simulink model "game"  (R2021a)
settings: Solver=VariableStepAuto  StartTime=0.0  StopTime=inf  RelTol=1e-3
libraries: vrlib x2
settings Model: Creator=kbhar  LastModifiedBy=kbhar

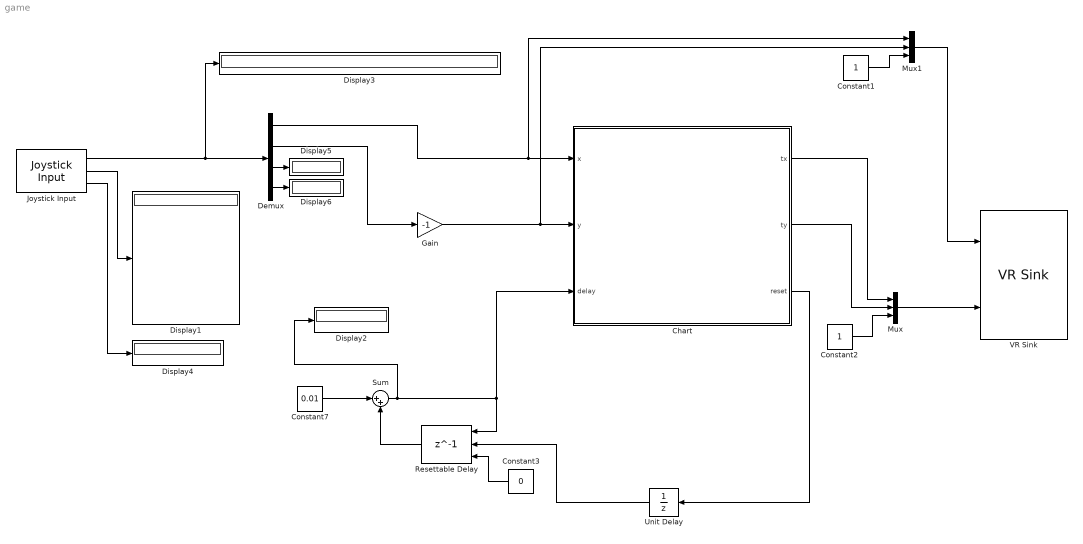
== system game ==
  Chart : Stateflow chart  TreatAsAtomicUnit=on
      settings: PortSchema="{\"entries\":[{\"content\":{\"sides\":[{\"content\":{\"connectorIds\":[\"In2\",\"In3\",\"In1\"]},\"type\":\"ConnectorPlacement.EquallySpacedRectSide\",\"uuid\":\"f1ac4276-d975-44f7-8e33-a85bf0c84183\"},{\"content\":{\"connectorIds\":[\"Out1\",\"Out2\",\"Out3\"],\"side\":\"RIGHT\"},\"type\":\"ConnectorPlacement.EquallySpacedRectSide\",\"uuid\":\"fad27161-645b-4edf-96e2-08eec94c36d6\"},{\"content\":{\"connectorIds\":[],\"side\":\"TOP\"},\"type\":\"ConnectorPlacement.EquallySpacedRectSide\",\"uuid\":\"b77dfb51-8030-4063-824e-9da8b3bcfc4a\"}]},\"type\":\"ConnectorPlacement.EquallySpacedConnector\",\"uuid\":\"85b5c07b-9026-46b4-be3f-3c9b0e47e395\"}],\"packageUris\":[\"http://schema.mathworks.com/mf0/Connector/R2020b\"],\"version\":\"1.0\"}"
  Constant1 : Constant
  Constant2 : Constant
  Constant3 : Constant  Value=0
  Constant7 : Constant  Value=0.01
  Demux : Demux
  Display{1..6} (6 alike) : Display
  Gain : Gain  Gain=-1
  Joystick Input : vrlib/Joystick Input  joyid=1  adjustports=on  forcefeed=off
  Mux : Mux  Inputs=3
  Mux1 : Mux  Inputs=3
  Resettable Delay : Delay  DelayLength=1  InitialConditionSource=Input port  ExternalReset=Rising
      settings: InputPortMap=u0,r5,p4
  Sum : Sum  Inputs=|++
  Unit Delay : UnitDelay  SampleTime=-1  HasFrameUpgradeWarning=on
  VR Sink : vrlib/VR Sink  InstantiateOnLoad=on  SampleTime=0.1  ViewEnable=on  RemoteChange=off  RemoteView=off  FieldsWritten=cursor.translation.3.1.1.double#target.translation.3.1.1.double  WorldFileName=game.wrl  AutoView=off  VideoDimensions=[]  AllowVariableSize=off  FigureProperties="{'Position', 'Name', 'Viewpoint', 'CameraBound', 'CameraDirection', 'CameraPosition', 'CameraUpVector', 'ZoomFactor', 'Antialiasing', 'Headlight', 'Lighting', 'NavPanel', 'Sound', 'StatusBar', 'Stereo3D', 'Stereo3DCameraOffset', 'Stereo3DHIT', 'ToolBar', 'Textures', 'Transparency', 'Triad', 'Wireframe', 'NavZones', 'NavMode', 'NavSpeed', 'CaptureFileFormat', 'CaptureFileName', 'Record2DCompressMethod', 'Record2DCompressQuality', 'Record2D', 'Record2DFileName', 'Record2DFPS'; [7.8340000000000009e+02   2.7179999999999995e+02   5.7600000000000000e+02   3.5000000000000000e+02], '', '', 'on', [-1.1111111570273457e-04   0.0000000000000000e+00  -9.9999999382716009e-01], [-2.1809524624175411e-04   5.2244997024536133e-01   8.0371428770549223e+00], [0.0000000000000000e+00   1.0000000000000000e+00   0.0000000000000000e+00], [1.0000000000000000e+00], 'on', 'on', 'on', 'halfbar', 'on', 'on', 'off', [1.0000000149011612e-01], [0.0000000000000000e+00], 'on', 'on', 'on', 'none', 'off', 'off', 'fly', 'normal', 'tif', '%f_anim_%n.tif', 'auto', [7.5000000000000000e+01], 'off', '%f_anim_%n.avi', 'auto'}"
  wires:
  Resettable Delay/1 -> Sum/2
  Constant7/1 -> Sum/1
  Sum/1 -> Display2/1, Resettable Delay/1, Chart/1(delay)
  Chart/3(reset) -> Unit Delay/1
  Unit Delay/1 -> Resettable Delay/2
  Chart/1(tx) -> Mux/1
  Chart/2(ty) -> Mux/2
  Mux/1 -> VR Sink/2
  Constant2/1 -> Mux/3
  Joystick Input/2 -> Display1/1
  Joystick Input/1 -> Display3/1, Demux/1
  Demux/1 -> Mux1/1, Chart/2(x)
  Demux/2 -> Gain/1
  Gain/1 -> Mux1/2, Chart/3(y)
  Constant1/1 -> Mux1/3
  Mux1/1 -> VR Sink/1
  Joystick Input/3 -> Display4/1
  Demux/3 -> Display5/1
  Demux/4 -> Display6/1
  Constant3/1 -> Resettable Delay/3

== stateflow chart game/Chart ==
  state startstate1
    tx = 0; ty = 0; reset = 0;
  state tempstate1
    reset = 0;
    temp = randi(4);
  state rightstate1
    tx = 1; ty = 0; reset = 0;
  state leftstate1
    tx = -1; ty = 0; reset = 0;
  state downstate1
    tx = 0; ty = -1; reset = 0;
  state upstate1
    tx = 0; ty = 1; reset = 0;
  state resetstate1
    reset = 1;
  (default) -> startstate1
  startstate1 -> tempstate1
  resetstate1 -> tempstate1
  tempstate1 -> rightstate1 [order 1] : [temp == 1]
  tempstate1 -> leftstate1 [order 2] : [temp == 2]
  tempstate1 -> downstate1 [order 3] : [temp == 3]
  tempstate1 -> upstate1 [order 4] : [temp == 4]
  rightstate1 -> resetstate1 : [delay>15 | (x == 1 & y == 0)]
  leftstate1 -> resetstate1 : [delay>15 | (x == -1 & y == 0)]
  downstate1 -> resetstate1 : [delay>15 | (x == 0 & y == -1)]
  upstate1 -> resetstate1 : [delay>15 | (x == 0 & y == 1)]
  data: delay input; x input; y input; tx output; ty output; reset output; temp local
